simulink model "DIGITAL_LQG_LTR_QUAD_TANK"  (R2014a)
settings: Solver=ode45  SolverMode=SingleTasking  StartTime=0.0  StopTime=t_run  RelTol=1e-3
values from neighbouring files (symbols this model uses):
  area_maior = pi*(d_maior.^2)/4    [Model.m]
  area_menor = pi*(d_menor.^2)/4    [Model.m]
  g = 980    [LQG_LTR_fen.m]    (also in LQG_LTR_ident.m; LQG_LTR_pheno.m; Model.m = 981)
  gamma = [0.55 0.54]    [Barreiras.m]    (also in Barriers.m)
  hinicial = [9 7 0 0]    [LQG_LTR_fen.m]    (also in LQG_LTR_ident.m; LQG_LTR_pheno.m; Model.m = [hi1 hi2 0 0])
  k = [18 18]    [Barreiras.m]    (also in Barriers.m)
  Kc11z = Kc(1,1).num{1,1}    [LQG_LTR_fen.m]    (also in LQG_LTR_ident.m; LQG_LTR_pheno.m)
  Kc12z = Kc(1,2).num{1,1}    [LQG_LTR_fen.m]    (also in LQG_LTR_ident.m; LQG_LTR_pheno.m)
  Kc21z = Kc(2,1).num{1,1}    [LQG_LTR_fen.m]    (also in LQG_LTR_ident.m; LQG_LTR_pheno.m)
  Kc22z = Kc(2,2).num{1,1}    [LQG_LTR_fen.m]    (also in LQG_LTR_ident.m; LQG_LTR_pheno.m)
  Kcp = Kc(1,1).den{1,1}    [LQG_LTR_fen.m]    (also in LQG_LTR_ident.m; LQG_LTR_pheno.m)
  Ts = 0.1    [LQG_LTR_fen.m]    (also in LQG_LTR_ident.m; LQG_LTR_pheno.m)
settings Model: Creator=matheus  LastModifiedBy=PLANTA_02
settings DataIOCC: SignalLoggingSaveFormat=ModelDataLogs
settings OptimizationCC: ExpressionDepthLimit=2147483647  SimCompilerOptimization=off
settings DebuggingCC: UnderspecifiedInitializationDetection=Classic  FcnCallInpInsideContextMsg=EnableAllAsWarning  FrameProcessingCompatibilityMsg=error  StateNameClashWarn=warning
settings RTWCC: RTWCompilerOptimization=off
settings GRTTargetCC: CombineOutputUpdateFcns=off  GRTInterface=on

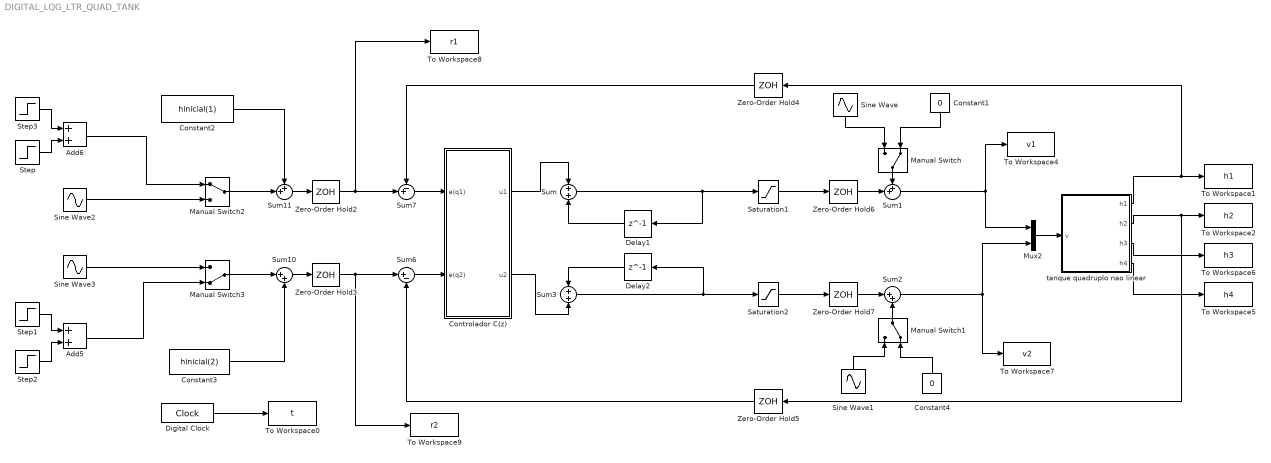
== system DIGITAL_LQG_LTR_QUAD_TANK ==
  Add5 : Sum
  Add6 : Sum
  Constant1 : Constant  Value=0
  Constant2 : Constant  Value=hinicial(1)
  Constant3 : Constant  Value=hinicial(2)
  Constant4 : Constant  Value=0
  Controlador C(z) : Subsystem
  Delay1 : Delay  DelayLength=1  InitialCondition=0  SampleTime=Ts
  Delay2 : Delay  DelayLength=1  InitialCondition=0  SampleTime=Ts
  Digital Clock : DigitalClock  SampleTime=Ts
  Manual Switch : ManualSwitch  CurrentSetting=0
  Manual Switch1 : ManualSwitch  CurrentSetting=0
  Manual Switch2 : ManualSwitch
  Manual Switch3 : ManualSwitch  CurrentSetting=0
  Mux2 : Mux  Inputs=2
  Saturation1 : Saturate  UpperLimit=10  LowerLimit=0
  Saturation2 : Saturate  UpperLimit=10  LowerLimit=0
  Sine Wave : Sin  Frequency=0.5  SampleTime=0
  Sine Wave1 : Sin  Frequency=0.5  Phase=pi/2  SampleTime=0
  Sine Wave2 : Sin  Frequency=0.1  SampleTime=0
  Sine Wave3 : Sin  Frequency=0.1  Phase=pi/2  SampleTime=0
  Step : Step  Time=400  After=-3  SampleTime=0  ZeroCross=off
  Step1 : Step  Time=200  After=3  SampleTime=0  ZeroCross=off
  Step2 : Step  Time=600  After=-3  SampleTime=0  ZeroCross=off
  Step3 : Step  Time=10  After=3  SampleTime=0  ZeroCross=off
  Sum : Sum
  Sum1 : Sum  Inputs=++|
  Sum10 : Sum  Inputs=|++
  Sum11 : Sum  Inputs=++|
  Sum2 : Sum  Inputs=|++
  Sum3 : Sum
  Sum6 : Sum  Inputs=|+-
  Sum7 : Sum  Inputs=-+|
  To Workspace0 : ToWorkspace  VariableName=t  SampleTime=-1
  To Workspace1 : ToWorkspace  VariableName=h1  SampleTime=-1
  To Workspace2 : ToWorkspace  VariableName=h2  SampleTime=-1
  To Workspace4 : ToWorkspace  VariableName=v1  SampleTime=-1
  To Workspace5 : ToWorkspace  VariableName=h4  SampleTime=-1
  To Workspace6 : ToWorkspace  VariableName=h3  SampleTime=-1
  To Workspace7 : ToWorkspace  VariableName=v2  SampleTime=-1
  To Workspace8 : ToWorkspace  VariableName=r1  SampleTime=-1
  To Workspace9 : ToWorkspace  VariableName=r2  SampleTime=-1
  Zero-Order Hold{2..7} (6 alike) : ZeroOrderHold  SampleTime=Ts
  tanque quadruplo nao linear : Subsystem
  wires:
  tanque quadruplo nao linear/1(h1) -> To Workspace1/1, Zero-Order Hold4/1
  tanque quadruplo nao linear/2(h2) -> To Workspace2/1, Zero-Order Hold5/1
  Mux2/1 -> tanque quadruplo nao linear/1(v)
  tanque quadruplo nao linear/4(h4) -> To Workspace5/1
  tanque quadruplo nao linear/3(h3) -> To Workspace6/1
  Sum10/1 -> Zero-Order Hold3/1
  Constant3/1 -> Sum10/2
  Step/1 -> Add6/2
  Step3/1 -> Add6/1
  Constant2/1 -> Sum11/1
  Step1/1 -> Add5/1
  Step2/1 -> Add5/2
  Sum11/1 -> Zero-Order Hold2/1
  Sum7/1 -> Controlador C(z)/1(e(q1))
  Sum6/1 -> Controlador C(z)/2(e(q2))
  Zero-Order Hold2/1 -> To Workspace8/1, Sum7/2
  Zero-Order Hold3/1 -> To Workspace9/1, Sum6/1
  Zero-Order Hold4/1 -> Sum7/1
  Zero-Order Hold5/1 -> Sum6/2
  Digital Clock/1 -> To Workspace0/1
  Sine Wave/1 -> Manual Switch/1
  Constant1/1 -> Manual Switch/2
  Sine Wave1/1 -> Manual Switch1/1
  Constant4/1 -> Manual Switch1/2
  Manual Switch/1 -> Sum1/1
  Sum1/1 -> To Workspace4/1, Mux2/1
  Manual Switch1/1 -> Sum2/2
  Sum2/1 -> To Workspace7/1, Mux2/2
  Add6/1 -> Manual Switch2/1
  Sine Wave2/1 -> Manual Switch2/2
  Sine Wave3/1 -> Manual Switch3/1
  Add5/1 -> Manual Switch3/2
  Manual Switch3/1 -> Sum10/1
  Manual Switch2/1 -> Sum11/2
  Sum/1 -> Delay1/1, Saturation1/1
  Sum3/1 -> Saturation2/1, Delay2/1
  Saturation1/1 -> Zero-Order Hold6/1
  Zero-Order Hold6/1 -> Sum1/2
  Saturation2/1 -> Zero-Order Hold7/1
  Zero-Order Hold7/1 -> Sum2/1
  Delay2/1 -> Sum3/1
  Controlador C(z)/2(u2) -> Sum3/2
  Controlador C(z)/1(u1) -> Sum/1
  Delay1/1 -> Sum/2

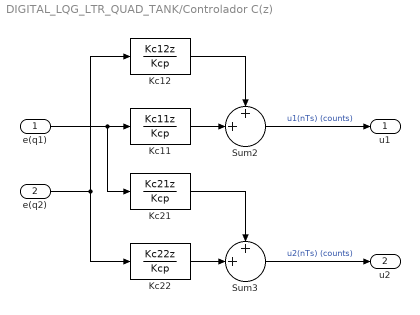
== system DIGITAL_LQG_LTR_QUAD_TANK/Controlador C(z) ==
  e(q1) : Inport
  e(q2) : Inport  Port=2
  Kc11 : DiscreteTransferFcn  Numerator=Kc11z  Denominator=Kcp  SampleTime=Ts
  Kc12 : DiscreteTransferFcn  Numerator=Kc12z  Denominator=Kcp  SampleTime=Ts
  Kc21 : DiscreteTransferFcn  Numerator=Kc21z  Denominator=Kcp  SampleTime=Ts
  Kc22 : DiscreteTransferFcn  Numerator=Kc22z  Denominator=Kcp  SampleTime=Ts
  Sum2 : Sum  Inputs=++|  SaturateOnIntegerOverflow=on  InputSameDT=on  OutDataTypeStr=Inherit: Same as first input
  Sum3 : Sum  Inputs=++|  SaturateOnIntegerOverflow=on  InputSameDT=on  OutDataTypeStr=Inherit: Same as first input
  u1 : Outport
  u2 : Outport  Port=2
  wires:
  e(q1)/1 -> Kc21/1, Kc11/1
  Kc11/1 -> Sum2/2
  e(q2)/1 -> Kc12/1, Kc22/1
  Kc22/1 -> Sum3/2
  Kc12/1 -> Sum2/1
  Kc21/1 -> Sum3/1
  Sum2/1 -> u1/1  "u1(nTs) (counts)"
  Sum3/1 -> u2/1  "u2(nTs) (counts)"

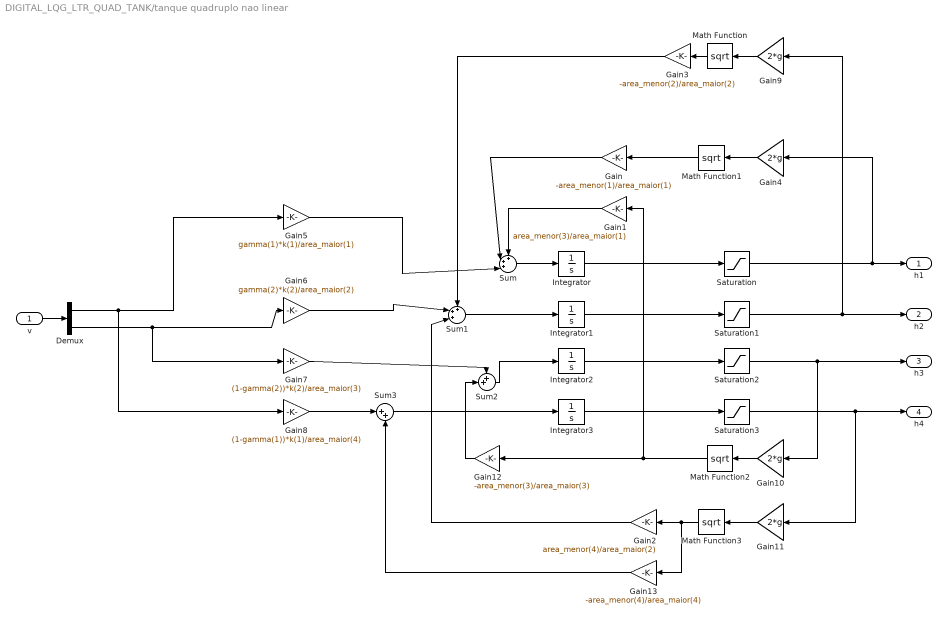
== system DIGITAL_LQG_LTR_QUAD_TANK/tanque quadruplo nao linear ==
  v : Inport
  Demux : Demux  Outputs=2
  Gain : Gain  Gain=-area_menor(1)/area_maior(1)
  Gain1 : Gain  Gain=area_menor(3)/area_maior(1)
  Gain{4,9..11} (4 alike) : Gain  Gain=2*g
  Gain12 : Gain  Gain=-area_menor(3)/area_maior(3)
  Gain13 : Gain  Gain=-area_menor(4)/area_maior(4)
  Gain2 : Gain  Gain=area_menor(4)/area_maior(2)
  Gain3 : Gain  Gain=-area_menor(2)/area_maior(2)
  Gain5 : Gain  Gain=gamma(1)*k(1)/area_maior(1)
  Gain6 : Gain  Gain=gamma(2)*k(2)/area_maior(2)
  Gain7 : Gain  Gain=(1-gamma(2))*k(2)/area_maior(3)
  Gain8 : Gain  Gain=(1-gamma(1))*k(1)/area_maior(4)
  Integrator : Integrator  InitialCondition=hinicial(1)
  Integrator1 : Integrator  InitialCondition=hinicial(2)
  Integrator2 : Integrator  InitialCondition=hinicial(3)
  Integrator3 : Integrator  InitialCondition=hinicial(4)
  Math Function{,1..3} (4 alike) : Math  Operator=sqrt  SaturateOnIntegerOverflow=on
  Saturation{,1..3} (4 alike) : Saturate  UpperLimit=30  LowerLimit=0
  Sum : Sum  Inputs=+++|
  Sum1 : Sum  Inputs=+++|
  Sum2 : Sum  Inputs=++|
  Sum3 : Sum  Inputs=|++
  h1 : Outport
  h2 : Outport  Port=2
  h3 : Outport  Port=3
  h4 : Outport  Port=4
  wires:
  v/1 -> Demux/1
  Integrator1/1 -> Saturation1/1
  Integrator3/1 -> Saturation3/1
  Integrator/1 -> Saturation/1
  Demux/1 -> Gain8/1, Gain5/1
  Sum/1 -> Integrator/1
  Gain1/1 -> Sum/1
  Gain/1 -> Sum/2
  Gain5/1 -> Sum/3
  Demux/2 -> Gain6/1, Gain7/1
  Sum1/1 -> Integrator1/1
  Gain4/1 -> Math Function1/1
  Gain9/1 -> Math Function/1
  Gain10/1 -> Math Function2/1
  Gain11/1 -> Math Function3/1
  Integrator2/1 -> Saturation2/1
  Gain3/1 -> Sum1/1
  Gain6/1 -> Sum1/2
  Gain2/1 -> Sum1/3
  Sum2/1 -> Integrator2/1
  Sum3/1 -> Integrator3/1
  Gain7/1 -> Sum2/1
  Gain12/1 -> Sum2/2
  Gain13/1 -> Sum3/2
  Gain8/1 -> Sum3/1
  Math Function/1 -> Gain3/1
  Math Function1/1 -> Gain/1
  Math Function2/1 -> Gain1/1, Gain12/1
  Math Function3/1 -> Gain2/1, Gain13/1
  Saturation/1 -> h1/1, Gain4/1
  Saturation1/1 -> h2/1, Gain9/1
  Saturation2/1 -> h3/1, Gain10/1
  Saturation3/1 -> h4/1, Gain11/1
